simulink model "exercise1_cours"  (Simulink 8.9)
settings: Solver=ode15s  StartTime=0.0  StopTime=10.0  RelTol=1e-6
undefined symbols (not defined in the file or in its folder): a, delta, Kprime, omega, omegah, omegal
settings Model: SuppressorTable=22 serialization::archive 11 0 6 0 0 0 0 0  Creator=martinguay  LastModifiedBy=martinguay
settings DataIOCC: LimitDataPoints=off  SaveFormat=Dataset  SignalLoggingSaveFormat=Dataset
settings OptimizationCC: LifeSpan=auto
settings DebuggingCC: UnderspecifiedInitializationDetection=Simplified  MergeDetectMultiDrivingBlocksExec=error  FcnCallInpInsideContextMsg=error  StateNameClashWarn=none  SFUnexpectedBacktrackingDiag=error  SFNoUnconditionalDefaultTransitionDiag=error  SFExecutionAtInitializationDiag=warning
settings HardwareCC: ProdBitPerPointer=64  ProdBitPerSizeT=64  ProdBitPerPtrDiffT=64  ProdLargestAtomicFloat=Float  ProdIntDivRoundTo=Zero  ProdEndianess=LittleEndian  ProdWordSize=64  ProdHWDeviceType=Intel->x86-64 (Windows64)
settings ModelReferenceCC: PropagateSignalLabelsOutOfModel=on
settings GRTTargetCC: TargetLangStandard=C99 (ISO)  GeneratePreprocessorConditionals=Use local settings  CombineOutputUpdateFcns=on  GRTInterface=off
settings ConfigComp: CovMetricSettings=dwe  CovHtmlReporting=off  CovSaveCumulativeToWorkspaceVar=off  CovSaveSingleToWorkspaceVar=off  CovExternalEMLEnable=on

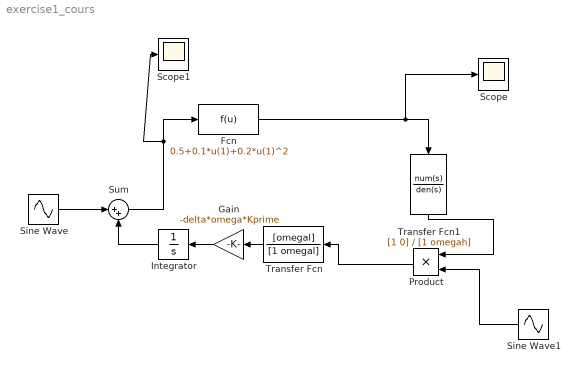
== system exercise1_cours ==
  Fcn : Fcn  Expr=0.5+0.1*u(1)+0.2*u(1)^2
  Gain : Gain  Gain=-delta*omega*Kprime
  Integrator : Integrator
  Product : Product
  Scope : Scope
  Scope1 : Scope
  Sine Wave : Sin  Amplitude=a  Frequency=omega  SampleTime=0
  Sine Wave1 : Sin  Amplitude=1/a  Frequency=omega  SampleTime=0
  Sum : Sum  Inputs=|++
  Transfer Fcn : TransferFcn  Numerator=[omegal]  Denominator=[1 omegal]
  Transfer Fcn1 : TransferFcn  Numerator=[1 0]  Denominator=[1 omegah]
  wires:
  Sine Wave/1 -> Sum/1
  Transfer Fcn/1 -> Gain/1
  Sum/1 -> Scope1/1, Fcn/1
  Sine Wave1/1 -> Product/2
  Transfer Fcn1/1 -> Product/1
  Product/1 -> Transfer Fcn/1
  Fcn/1 -> Scope/1, Transfer Fcn1/1
  Gain/1 -> Integrator/1
  Integrator/1 -> Sum/2
